simulink model "HDLExampleCosim"  (R2024a)
settings: Solver=FixedStepDiscrete  StartTime=0.0  StopTime=simTime  RelTol=1e-3
values from neighbouring files (symbols this model uses):
  sampleTime = 1    [exampleCosim.m]
libraries: dspsrcs4 x1
settings Model: DataTypeOverride=Off  Creator=cotti  LastModifiedBy=cotti
settings OptimizationCC: BlockReduction=off  ConditionallyExecuteInputs=off  DefaultParameterBehavior=Inlined  InheritOutputTypeSmallerThanSingle=on  ReuseModelBlockBuffer=off
settings DebuggingCC: AlgebraicLoopMsg=error  SingleTaskRateTransMsg=error
settings HardwareCC: ProdBitPerPointer=32  ProdBitPerSizeT=32  ProdBitPerPtrDiffT=32  ProdLargestAtomicFloat=None  ProdIntDivRoundTo=Undefined  ProdEndianess=Unspecified  ProdWordSize=32  ProdHWDeviceType=ASIC/FPGA->ASIC/FPGA  TargetBitPerLong=64  TargetBitPerPointer=64  TargetBitPerSizeT=64  TargetBitPerPtrDiffT=64  TargetLongLongMode=on  TargetIntDivRoundTo=Zero  TargetEndianess=LittleEndian  TargetWordSize=64  TargetHWDeviceType=Custom Processor->MATLAB Host Computer  ProdEqTarget=off
settings RTWCC: GPUComputeCapability=3.5

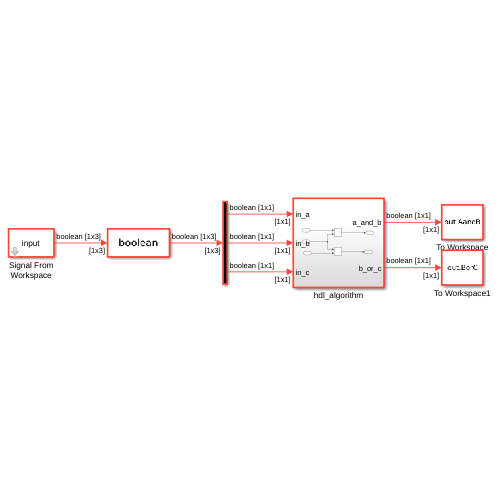
[thumbnail: Simulink's stored preview of the top-level diagram]
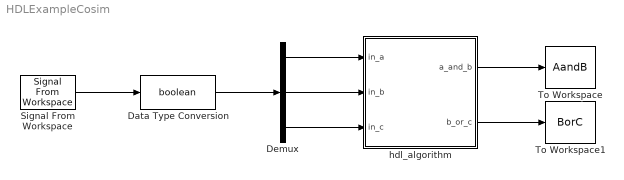
== system HDLExampleCosim ==
  Data Type Conversion : DataTypeConversion  OutDataTypeStr=boolean  SaturateOnIntegerOverflow=off  RndMeth=Floor
  Demux : Demux  Outputs=3
  Signal From Workspace : dspsrcs4/Signal From Workspace  X=input  Ts=sampleTime  nsamps=sampleSize  OutputAfterFinalValue=Setting to zero  ignoreOrWarnInputAndFrameLengths=off  OutputFrames=off
  To Workspace : ToWorkspace  VariableName=AandB  SaveFormat=Timeseries  SampleTime=-1
      settings: Save2DSignal=2-D array (concatenate along first dimension)
  To Workspace1 : ToWorkspace  VariableName=BorC  SaveFormat=Timeseries  SampleTime=-1
      settings: Save2DSignal=2-D array (concatenate along first dimension)
  hdl_algorithm : Subsystem
  wires:
  Demux/3 -> hdl_algorithm/3(in_c)
  Demux/2 -> hdl_algorithm/2(in_b)
  Demux/1 -> hdl_algorithm/1(in_a)
  Signal From Workspace/1 -> Data Type Conversion/1
  Data Type Conversion/1 -> Demux/1
  hdl_algorithm/1(a_and_b) -> To Workspace/1
  hdl_algorithm/2(b_or_c) -> To Workspace1/1

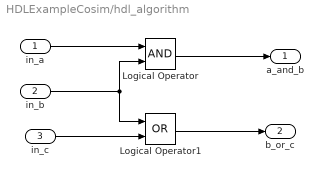
== system HDLExampleCosim/hdl_algorithm ==
  in_a : Inport
  in_b : Inport  Port=2
  in_c : Inport  Port=3
  Logical Operator : Logic  AllPortsSameDT=off  OutDataTypeStr=boolean
  Logical Operator1 : Logic  Operator=OR  AllPortsSameDT=off  OutDataTypeStr=boolean
  a_and_b : Outport
  b_or_c : Outport  Port=2
  wires:
  Logical Operator/1 -> a_and_b/1
  in_a/1 -> Logical Operator/1
  in_b/1 -> Logical Operator1/1, Logical Operator/2
  in_c/1 -> Logical Operator1/2
  Logical Operator1/1 -> b_or_c/1
